simulink model "dbs_ut"  (Simulink 8.1)
settings: Solver=FixedStepDiscrete  StartTime=0.0  StopTime=50  FixedStep=5e-3  RelTol=1e-3
libraries: siltestlib x6, dbs x1, hcu_lib x1
settings Model: Creator=xsellart  LastModifiedBy=tescamilla
settings DataIOCC: SignalLoggingSaveFormat=Dataset
settings OptimizationCC: ExpressionDepthLimit=128
settings DebuggingCC: FcnCallInpInsideContextMsg=EnableAllAsError
settings GRTTargetCC: CombineOutputUpdateFcns=on  GRTInterface=off

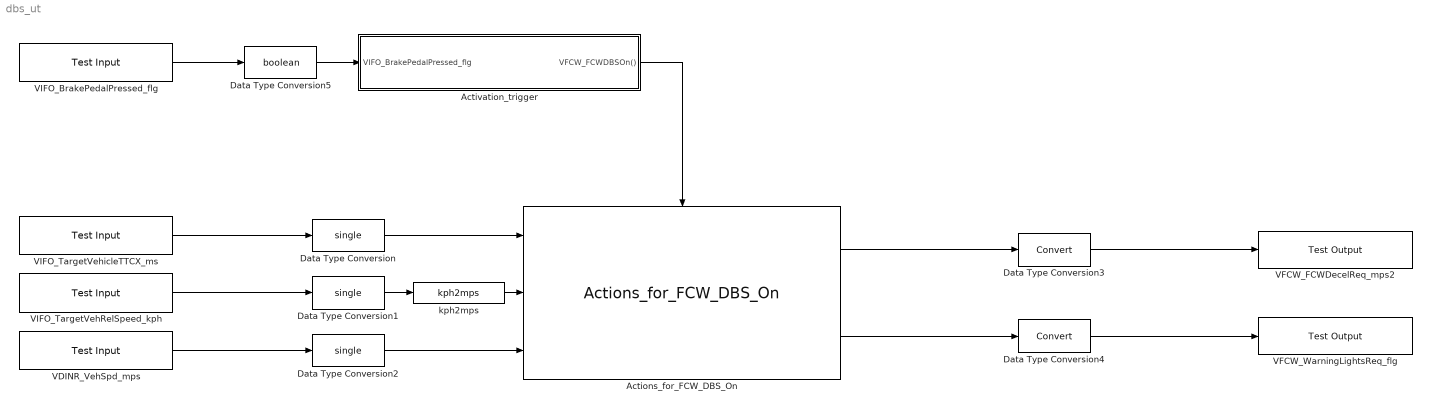
== system dbs_ut ==
  Actions_for_FCW_DBS_On : dbs/Actions_for_FCW_DBS_On
  Activation_trigger : Stateflow chart  TreatAsAtomicUnit=on
  Data Type Conversion : DataTypeConversion  OutDataTypeStr=single
  Data Type Conversion1 : DataTypeConversion  OutDataTypeStr=single
  Data Type Conversion2 : DataTypeConversion  OutDataTypeStr=single
  Data Type Conversion3 : DataTypeConversion
  Data Type Conversion4 : DataTypeConversion
  Data Type Conversion5 : DataTypeConversion  OutDataTypeStr=boolean
  VDINR_VehSpd_mps : siltestlib/Test Input  varname=VDINR_VehSpd_mps  sampletime=-1
  VFCW_FCWDecelReq_mps2 : siltestlib/Test Output  varname=VFCW_FCWDecelReq_mps2  sampletime=-1
  VFCW_WarningLightsReq_flg : siltestlib/Test Output  varname=VFCW_WarningLightsReq_flg  sampletime=-1
  VIFO_BrakePedalPressed_flg : siltestlib/Test Input  varname=VIFO_BrakePedalPressed_flg  sampletime=-1
  VIFO_TargetVehRelSpeed_kph : siltestlib/Test Input  varname=VIFO_TargetVehRelSpeed_kph  sampletime=-1
  VIFO_TargetVehicleTTCX_ms : siltestlib/Test Input  varname=VIFO_TargetVehicleTTCX_ms  sampletime=-1
  kph2mps : hcu_lib/kph2mps
  wires:
  Activation_trigger/1(VFCW_FCWDBSOn()) -> Actions_for_FCW_DBS_On/Trigger
  VIFO_TargetVehicleTTCX_ms/1 -> Data Type Conversion/1
  VIFO_TargetVehRelSpeed_kph/1 -> Data Type Conversion1/1
  VDINR_VehSpd_mps/1 -> Data Type Conversion2/1
  Data Type Conversion/1 -> Actions_for_FCW_DBS_On/1
  Data Type Conversion1/1 -> kph2mps/1
  Data Type Conversion2/1 -> Actions_for_FCW_DBS_On/3
  Actions_for_FCW_DBS_On/1 -> Data Type Conversion3/1
  Data Type Conversion3/1 -> VFCW_FCWDecelReq_mps2/1
  Actions_for_FCW_DBS_On/2 -> Data Type Conversion4/1
  Data Type Conversion4/1 -> VFCW_WarningLightsReq_flg/1
  Data Type Conversion5/1 -> Activation_trigger/1(VIFO_BrakePedalPressed_flg)
  VIFO_BrakePedalPressed_flg/1 -> Data Type Conversion5/1
  kph2mps/1 -> Actions_for_FCW_DBS_On/2

== stateflow chart Activation_trigger ==
  state A
  state B
    bind: VFCW_FCWDBSOn;
    en:
    VFCW_FCWDBSOn;
    du:
    VFCW_FCWDBSOn;
  (default) -> A
  A -> B : [VIFO_BrakePedalPressed_flg == 1]
  B -> A : [VIFO_BrakePedalPressed_flg == 0]
  data: VIFO_BrakePedalPressed_flg input boolean
  events: VFCW_FCWDBSOn output FUNCTION_CALL_EVENT
